simulink model "PI_controller_windup_electrical"  (R2019b)
settings: Solver=FixedStepAuto  StartTime=0.0  StopTime=2  FixedStep=0.001  RelTol=1e-3
settings Model: Creator=suvo  LastModifiedBy=suvo

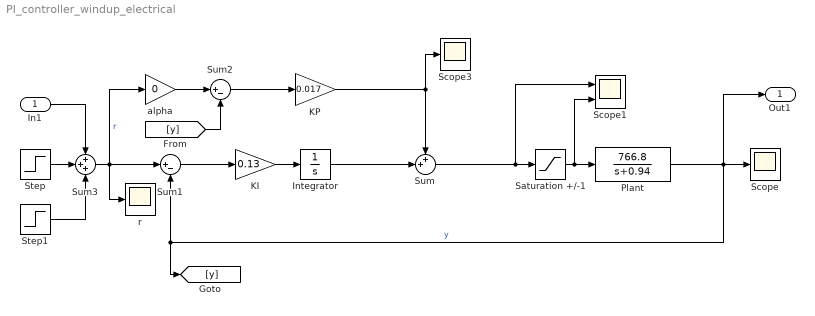
== system PI_controller_windup_electrical ==
  In1 : Inport
  Integrator : Integrator
  KI : Gain  Gain=0.13
  KP : Gain  Gain=0.017
  Plant : TransferFcn  Numerator=766.8  Denominator=[1 0.94]
  Saturation +/-1 : Saturate  UpperLimit=3  LowerLimit=0
  Scope : Scope
  Scope1 : Scope  NumInputPorts=2
  Scope3 : Scope
  Step : Step  Time=0  After=1000  SampleTime=0
  Step1 : Step  Time=3  After=0  SampleTime=0
  Sum : Sum  Inputs=++|
  Sum1 : Sum  Inputs=|+-
  Sum2 : Sum  Inputs=|+-
  Sum3 : Sum  Inputs=+++
  alpha : Gain  Gain=0
  r : Scope
  Out1 : Outport
  wires:
  KI/1 -> Integrator/1
  Sum1/1 -> KI/1
  Plant/1 -> Scope/1, Out1/1, Sum1/2, [y]  "y"
  Sum3/1 -> r/1, alpha/1, Sum1/1  "r"
  Sum2/1 -> KP/1
  KP/1 -> Sum/1, Scope3/1
  In1/1 -> Sum3/1
  Step/1 -> Sum3/2
  [y] -> Sum2/2
  alpha/1 -> Sum2/1
  Sum/1 -> Scope1/1, Saturation +/-1/1
  Saturation +/-1/1 -> Scope1/2, Plant/1
  Step1/1 -> Sum3/3
  Integrator/1 -> Sum/2
